simulink model "drone_5DOF"  (R2023b)
settings: Solver=ode45  StartTime=0.0  StopTime=1  FixedStep=0.0001  MaxStep=0.001  RelTol=1e-3
values from neighbouring files (symbols this model uses):
  A = [-qr-qu,0,0,0 ... (first row only)    [partA.m]    (also in partB.m = zeros(10,10))
  B = [1,0;0,0;0,1;0,0]    [partA.m]    (also in partB.m = zeros(10,3))
  g = 9.81    [droneStates.m]    (also in partB.m)
  K = place(A,B,[tau tau*2 tau tau*2])    [partA.m]    (also in partB.m = zeros(3,10))
  mass = 0.1    [droneStates.m]    (also in partB.m)
  stateNoiseGain = zeros(10,1)    [partB.m]
  stepVal = [0,0,0]    [partB.m]
  x0 = randn(n,1).*[1,1,0,1,1,1,0.1,0.1,0,0]'*1    [partB.m]
libraries: simulink x1, dspsrcs4 x1
settings Model: SimulationMode=rapid-accelerator  Creator=Shadow  LastModifiedBy=Shadow
settings OptimizationCC: DefaultUnderspecifiedDataType=single

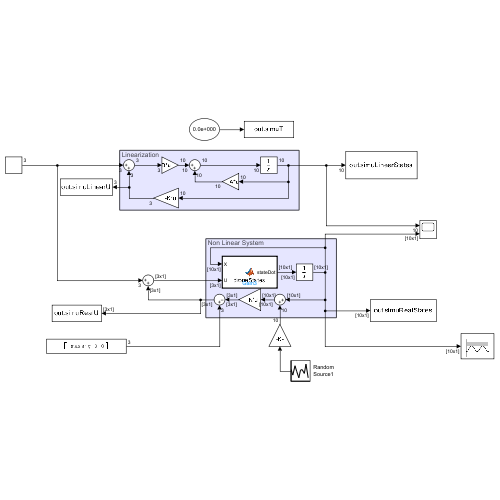
[thumbnail: Simulink's stored preview of the top-level diagram]
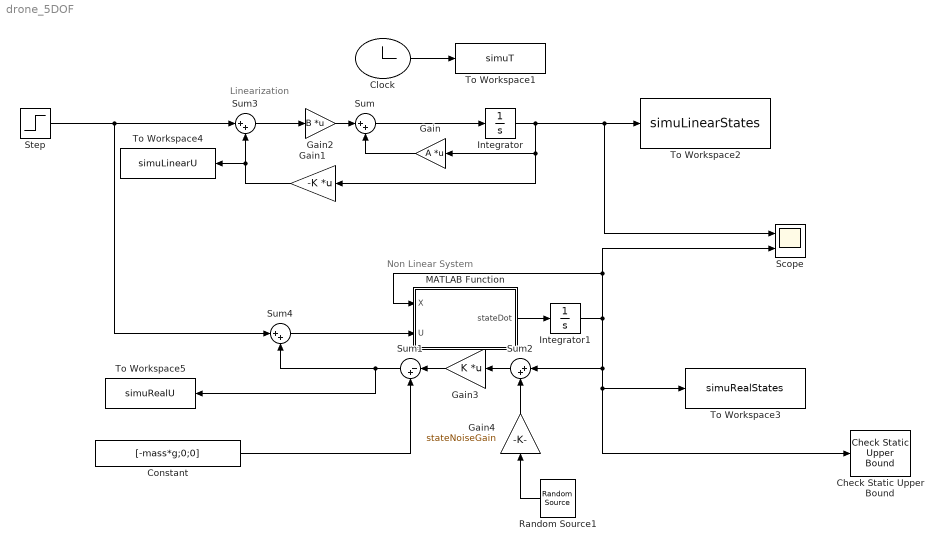
== system drone_5DOF ==
  note: Non Linear System
  note: Linearization
  Check Static Upper Bound : simulink/Model Verification/Check Static  Upper Bound  Description=u <= 1e10  max=1e10  max_included=on  enabled=on  stopWhenAssertionFail=on  export=off  icon=graphic
  Clock : Clock
  Constant : Constant  Value=[-mass*g;0;0]
  Gain : Gain  Gain=A  Multiplication=Matrix(K*u)
  Gain1 : Gain  Gain=-K  Multiplication=Matrix(K*u)
  Gain2 : Gain  Gain=B  Multiplication=Matrix(K*u)
  Gain3 : Gain  Gain=K  Multiplication=Matrix(K*u)
  Gain4 : Gain  Gain=stateNoiseGain
  Integrator : Integrator  InitialCondition=x0
  Integrator1 : Integrator  InitialCondition=x0
  MATLAB Function : MATLAB Function  TreatAsAtomicUnit=on
  Random Source1 : dspsrcs4/Random Source  SrcType=Gaussian  NormMethod=Ziggurat  CltLength=12  MinVal=0  MaxVal=1  MeanVal=0  VarVal=1  RepMode=Not repeatable  rawSeed=1  IsInherit=on  SampMode=Discrete  SampTime=1  SampFrame=1  DataType=Double  OutComplex=Real  OutputFrames=off
  Scope : Scope  NumInputPorts=2
  Step : Step  Time=0.1  After=stepVal  SampleTime=0
  Sum{,2..4} (4 alike) : Sum  Inputs=|++
  Sum1 : Sum  Inputs=|-+
  To Workspace1 : ToWorkspace  VariableName=simuT  SampleTime=0.01
      settings: Save2DSignal=2-D array (concatenate along first dimension)
  To Workspace2 : ToWorkspace  VariableName=simuLinearStates  SampleTime=0.01
      settings: Save2DSignal=2-D array (concatenate along first dimension)
  To Workspace3 : ToWorkspace  VariableName=simuRealStates  SampleTime=0.01
      settings: Save2DSignal=2-D array (concatenate along first dimension)
  To Workspace4 : ToWorkspace  VariableName=simuLinearU  SampleTime=0.01
      settings: Save2DSignal=2-D array (concatenate along first dimension)
  To Workspace5 : ToWorkspace  VariableName=simuRealU  SampleTime=0.01
      settings: Save2DSignal=2-D array (concatenate along first dimension)
  wires:
  Integrator/1 -> Scope/1, To Workspace2/1, Gain1/1, Gain/1
  Gain/1 -> Sum/2
  Gain2/1 -> Sum/1
  MATLAB Function/1(stateDot) -> Integrator1/1
  Integrator1/1 -> Sum2/1, To Workspace3/1, Check Static Upper Bound/1, Scope/2, MATLAB Function/1(X)
  Clock/1 -> To Workspace1/1
  Constant/1 -> Sum1/2
  Sum/1 -> Integrator/1
  Gain3/1 -> Sum1/1
  Sum1/1 -> Sum4/2, To Workspace5/1
  Gain1/1 -> To Workspace4/1, Sum3/2
  Sum3/1 -> Gain2/1
  Step/1 -> Sum4/1, Sum3/1
  Sum4/1 -> MATLAB Function/2(U)
  Gain4/1 -> Sum2/2
  Sum2/1 -> Gain3/1
  Random Source1/1 -> Gain4/1

== matlab function drone_5DOF/MATLAB Function ==
  data: X input size=10; stateDot output; U input size=3
function stateDot=droneStates(X,U)
g=9.81;
mass = 0.1;
Ix = 1e-4;
Iy = 1e-4;

x=X(1);
y=X(2);
z=X(3);
xdot=X(4);
ydot=X(5);
zdot=X(6);
phi=X(7);
theta=X(8);
phidot=X(9);
thetadot=X(10);
ft=U(1);
taux=U(2);
tauy=U(3);



stateDot=[xdot;
    ydot; 
    zdot;
    -thetadot*zdot-g*sin(theta);
    phidot*zdot+g*cos(theta)*sin(phi);
    thetadot*xdot-phidot*ydot+g*cos(theta)*cos(phi)-ft/mass;
    phidot;
    thetadot;
    taux/Ix;
    tauy/Iy];
% 
% stateDot=[xdot;
%     ydot; 
%     zdot;
%     -ft/mass*cos(phi)*sin(theta);
%     ft/mass*sin(theta);
%     g-ft/mass*(cos(phi)*cos(theta));
%     phidot;
%     thetadot;    
%     taux/Ix;
%     tauy/Iy];
